simulink model "ModeloUnaOrugaFCVisibles"  (R2023b)
(part 3 of 16)

  Connection Label384/LConn1 -- Simscape Bus3/LConn5
  Connection Label309/LConn1 -- Simscape Bus2/LConn31
  Simscape Bus3/LConn16 -- Connection Label361/LConn1
  Connection Label364/LConn1 -- Simscape Bus3/LConn10
  Connection Label325/LConn1 -- Simscape Bus2/LConn17
  Connection Label342/LConn1 -- Simscape Bus3/LConn43
  Connection Label365/LConn1 -- Simscape Bus3/LConn28
  Connection Label345/LConn1 -- Simscape Bus3/LConn40
  Connection Label354/LConn1 -- Simscape Bus3/LConn31
  Connection Label315/LConn1 -- Simscape Bus2/LConn18
  Connection Label349/LConn1 -- Simscape Bus3/LConn36
  Connection Label338/LConn1 -- Simscape Bus2/LConn2
  Connection Label376/LConn1 -- Simscape Bus3/LConn25
  Simscape Bus3/LConn4 -- Connection Label381/LConn1
  Connection Label353/LConn1 -- Simscape Bus3/LConn32
  Simscape Bus2/LConn4 -- Connection Label337/LConn1
  Simscape Bus3/LConn24 -- Connection Label357/LConn1
  Connection Label323/LConn1 -- Simscape Bus2/LConn21
  Simscape Bus3/LConn8 -- Connection Label379/LConn1
  Connection Label331/LConn1 -- Simscape Bus2/LConn25
  Connection Label304/LConn1 -- Simscape Bus2/LConn36
  Simscape Bus2/LConn12 -- Connection Label318/LConn1
  Connection Label387/LConn1 -- Simscape Bus3/LConn47
  Connection Label308/LConn1 -- Simscape Bus2/LConn32
  Connection Label343/LConn1 -- Simscape Bus3/LConn42
  Simscape Bus3/LConn20 -- Connection Label359/LConn1
  Simscape Bus2/LConn8 -- Connection Label335/LConn1
  Connection Label341/LConn1 -- Simscape Bus2/LConn5
  Connection Label375/LConn1 -- Simscape Bus3/LConn27
  Connection Label317/LConn1 -- Simscape Bus2/LConn14
  Connection Label295/LConn1 -- Simscape Bus2/LConn45
  Simscape Bus3/LConn26 -- Connection Label366/LConn1
  Connection Label389/LConn1 -- Simscape Bus2/LConn49
  Simscape Bus2/LConn30 -- Connection Label310/LConn1
  Connection Label368/LConn1 -- Simscape Bus3/LConn21
  Connection Label356/LConn1 -- Simscape Bus3/LConn29
  Connection Label301/LConn1 -- Simscape Bus2/LConn39
  Connection Label367/LConn1 -- Simscape Bus3/LConn23
  Connection Label329/LConn1 -- Simscape Bus2/LConn9
  Connection Label298/LConn1 -- Simscape Bus2/LConn42
  Simscape Bus2/LConn22 -- Connection Label313/LConn1
  Connection Label322/LConn1 -- Simscape Bus2/LConn23
  Connection Label296/LConn1 -- Simscape Bus2/LConn44
  Connection Label374/LConn1 -- Simscape Bus3/LConn9
  Connection Label352/LConn1 -- Simscape Bus3/LConn33
  Connection Label378/LConn1 -- Simscape Bus3/LConn1
  Simscape Bus3/LConn22 -- Connection Label358/LConn1
  Simscape Bus3/RConn1 -- AAP/RConn1
  Connection Label385/LConn1 -- Simscape Bus3/LConn49
  Simscape Bus2/RConn1 -- AA/RConn1
  Revolute Joint34/LConn1 -- Pieza_Correa_61_RIGID/RConn1
  Revolute Joint43/LConn1 -- Pieza_Correa_52_RIGID/RConn1
  Revolute Joint47/LConn1 -- Pieza_Correa_74_RIGID/LConn1
  Revolute Joint13/LConn1 -- Pieza_Correa_88_RIGID/RConn1
  Revolute Joint31/LConn1 -- Pieza_Correa_64_RIGID/RConn1
  Revolute Joint10/LConn1 -- Pieza_Correa_85_RIGID/RConn1
  Revolute Joint40/RConn1 -- Pieza_Correa_56_RIGID/LConn1
  Revolute Joint6/RConn1 -- Pieza_Correa_82_RIGID/LConn1
  Revolute Joint7/LConn1 -- Pieza_Correa_82_RIGID/RConn1
  Revolute Joint3/LConn1 -- Pieza_Correa_78_RIGID1/RConn1
  Revolute Joint46/RConn1 -- Pieza_Correa_50_RIGID/LConn1
  Revolute Joint37/LConn1 -- Pieza_Correa_58_RIGID/RConn1
  Revolute Joint16/RConn1 -- Pieza_Correa_92_RIGID/LConn1
  Revolute Joint3/RConn1 -- Pieza_Correa_79_RIGID/LConn1
  Revolute Joint25/RConn1 -- Pieza_Correa_71_RIGID/LConn1
  Revolute Joint21/LConn1 -- Pieza_Correa_96_RIGID/RConn1
  Revolute Joint48/RConn1 -- Pieza_Correa_90_RIGID/LConn1
  Revolute Joint14/LConn1 -- Pieza_Correa_97_RIGID/RConn1
  Revolute Joint24/LConn1 -- Pieza_Correa_71_RIGID/RConn1
  Revolute Joint43/RConn1 -- Pieza_Correa_53_RIGID/LConn1
  Revolute Joint28/RConn1 -- Pieza_Correa_68_RIGID/LConn1
  Revolute Joint/LConn1 -- Pieza_Correa_1_RIGID/LConn2
  Revolute Joint23/LConn1 -- Pieza_Correa_72_RIGID/RConn1
  Revolute Joint12/RConn1 -- Pieza_Correa_88_RIGID/LConn1
  Revolute Joint15/LConn1 -- Pieza_Correa_90_RIGID/RConn1
  Revolute Joint21/RConn1 -- Pieza_Correa_97_RIGID/LConn1
  Revolute Joint22/LConn1 -- Pieza_Correa_75_RIGID/LConn1
  Revolute Joint5/RConn1 -- Pieza_Correa_81_RIGID/LConn1
  Revolute Joint46/LConn1 -- Pieza_Correa_1_RIGID/RConn3
  Revolute Joint2/RConn1 -- Pieza_Correa_78_RIGID1/LConn1
  Revolute Joint16/LConn1 -- Pieza_Correa_91_RIGID/RConn1
  Revolute Joint11/LConn1 -- Pieza_Correa_86_RIGID/RConn1
  Revolute Joint48/LConn1 -- Pieza_Correa_89_RIGID/RConn1
  Revolute Joint23/RConn1 -- Pieza_Correa_73_RIGID/LConn1
  Revolute Joint11/RConn1 -- Pieza_Correa_87_RIGID/LConn1
  Revolute Joint39/LConn1 -- Pieza_Correa_56_RIGID/RConn1
  Revolute Joint18/RConn1 -- Pieza_Correa_94_RIGID/LConn1
  Revolute Joint4/RConn1 -- Pieza_Correa_80_RIGID/LConn1
  Revolute Joint12/LConn1 -- Pieza_Correa_87_RIGID/RConn1
  Revolute Joint26/RConn1 -- Pieza_Correa_70_RIGID/LConn1
  Revolute Joint5/LConn1 -- Pieza_Correa_80_RIGID/RConn1
  Revolute Joint34/RConn1 -- Pieza_Correa_62_RIGID/LConn1
  Revolute Joint30/RConn1 -- Pieza_Correa_66_RIGID/LConn1
  Revolute Joint33/LConn1 -- Pieza_Correa_62_RIGID/RConn1
  Revolute Joint20/RConn1 -- Pieza_Correa_96_RIGID/LConn1
  Revolute Joint27/RConn1 -- Pieza_Correa_69_RIGID/LConn1
  Revolute Joint37/RConn1 -- Pieza_Correa_59_RIGID/LConn1
  Revolute Joint15/RConn1 -- Pieza_Correa_91_RIGID/LConn1
  Revolute Joint19/LConn1 -- Pieza_Correa_94_RIGID/RConn1
  Revolute Joint1/RConn1 -- Pieza_Correa_77_RIGID/LConn1
  Revolute Joint8/LConn1 -- Pieza_Correa_83_RIGID/RConn1
  Revolute Joint20/LConn1 -- Pieza_Correa_95_RIGID/RConn1
  Revolute Joint24/RConn1 -- Pieza_Correa_72_RIGID/LConn1
  Revolute Joint7/RConn1 -- Pieza_Correa_83_RIGID/LConn1
  Revolute Joint41/LConn1 -- Pieza_Correa_54_RIGID/RConn1
  Revolute Joint29/RConn1 -- Pieza_Correa_67_RIGID/LConn1
  Revolute Joint17/LConn1 -- Pieza_Correa_92_RIGID/RConn1
  Pieza_Correa_73_RIGID/RConn1 -- Revolute Joint47/RConn1
  Revolute Joint36/RConn1 -- Pieza_Correa_60_RIGID/LConn1
  Revolute Joint13/RConn1 -- Pieza_Correa_89_RIGID/LConn1
  Revolute Joint8/RConn1 -- Pieza_Correa_84_RIGID/LConn1
  Revolute Joint22/RConn1 -- Pieza_Correa_74_RIGID/RConn1
  Revolute Joint26/LConn1 -- Pieza_Correa_69_RIGID/RConn1
  Revolute Joint10/RConn1 -- Pieza_Correa_86_RIGID/LConn1
  Revolute Joint40/LConn1 -- Pieza_Correa_55_RIGID/RConn1
  Revolute Joint36/LConn1 -- Pieza_Correa_59_RIGID/RConn1
  Revolute Joint39/RConn1 -- Pieza_Correa_57_RIGID/LConn1
  Revolute Joint14/RConn1 -- Pieza_Correa_75_RIGID/RConn1
  Revolute Joint35/LConn1 -- Pieza_Correa_60_RIGID/RConn1
  Revolute Joint33/RConn1 -- Pieza_Correa_63_RIGID/LConn1
  Revolute Joint38/LConn1 -- Pieza_Correa_57_RIGID/RConn1
  Revolute Joint31/RConn1 -- Pieza_Correa_65_RIGID/LConn1
  Revolute Joint38/RConn1 -- Pieza_Correa_58_RIGID/LConn1
  Revolute Joint42/RConn1 -- Pieza_Correa_54_RIGID/LConn1
  Revolute Joint35/RConn1 -- Pieza_Correa_61_RIGID/LConn1
  Revolute Joint32/RConn1 -- Pieza_Correa_64_RIGID/LConn1
  Revolute Joint45/LConn1 -- Pieza_Correa_50_RIGID/RConn1
  Revolute Joint44/RConn1 -- Pieza_Correa_52_RIGID/LConn1
  Revolute Joint17/RConn1 -- Pieza_Correa_93_RIGID/LConn1
  Revolute Joint2/LConn1 -- Pieza_Correa_77_RIGID/RConn1
  Revolute Joint6/LConn1 -- Pieza_Correa_81_RIGID/RConn1
  Revolute Joint29/LConn1 -- Pieza_Correa_66_RIGID/RConn1
  Revolute Joint28/LConn1 -- Pieza_Correa_67_RIGID/RConn1
  Revolute Joint4/LConn1 -- Pieza_Correa_79_RIGID/RConn1
  Revolute Joint/RConn1 -- Pieza_Correa_76_RIGID/LConn1
  Revolute Joint9/RConn1 -- Pieza_Correa_85_RIGID/LConn1
  Revolute Joint19/RConn1 -- Pieza_Correa_95_RIGID/LConn1
  Revolute Joint27/LConn1 -- Pieza_Correa_68_RIGID/RConn1
  Revolute Joint1/LConn1 -- Pieza_Correa_76_RIGID/RConn1
  Revolute Joint25/LConn1 -- Pieza_Correa_70_RIGID/RConn1
  Revolute Joint30/LConn1 -- Pieza_Correa_65_RIGID/RConn1
  Revolute Joint42/LConn1 -- Pieza_Correa_53_RIGID/RConn1
  Revolute Joint18/LConn1 -- Pieza_Correa_93_RIGID/RConn1
  Revolute Joint9/LConn1 -- Pieza_Correa_84_RIGID/RConn1
  Revolute Joint45/RConn1 -- Pieza_Correa_51_RIGID/LConn1
  Revolute Joint32/LConn1 -- Pieza_Correa_63_RIGID/RConn1
  Revolute Joint44/LConn1 -- Pieza_Correa_51_RIGID/RConn1
  Pieza_Correa_1_RIGID/RConn1 -- Connection Label8/LConn1
  Pieza_Correa_1_RIGID/RConn2 -- Connection Label12/LConn1
  Connection Label79/LConn1 -- Pieza_Correa_92_RIGID/LConn2
  Connection Label76/LConn1 -- Pieza_Correa_92_RIGID/LConn3
  Pieza_Correa_93_RIGID/LConn2 -- Connection Label83/LConn1
  Connection Label80/LConn1 -- Pieza_Correa_93_RIGID/LConn3
  Pieza_Correa_94_RIGID/LConn3 -- Connection Label84/LConn1
  Pieza_Correa_94_RIGID/LConn2 -- Connection Label87/LConn1
  Pieza_Correa_95_RIGID/LConn3 -- Connection Label88/LConn1
  Pieza_Correa_95_RIGID/LConn2 -- Connection Label91/LConn1
  Pieza_Correa_96_RIGID/LConn3 -- Connection Label92/LConn1
  Pieza_Correa_96_RIGID/LConn2 -- Connection Label95/LConn1
  Pieza_Correa_75_RIGID/LConn2 -- Connection Label100/LConn1
  Pieza_Correa_75_RIGID/LConn3 -- Connection Label103/LConn1
  Pieza_Correa_74_RIGID/LConn2 -- Connection Label104/LConn1
  Pieza_Correa_74_RIGID/LConn3 -- Connection Label107/LConn1
  Pieza_Correa_73_RIGID/LConn3 -- Connection Label108/LConn1
  Pieza_Correa_73_RIGID/LConn2 -- Connection Label111/LConn1
  Pieza_Correa_72_RIGID/LConn3 -- Connection Label112/LConn1
  Pieza_Correa_72_RIGID/LConn2 -- Connection Label115/LConn1
  Pieza_Correa_71_RIGID/LConn3 -- Connection Label116/LConn1
  Pieza_Correa_71_RIGID/LConn2 -- Connection Label119/LConn1
  Pieza_Correa_70_RIGID/LConn3 -- Connection Label120/LConn1
  Pieza_Correa_70_RIGID/LConn2 -- Connection Label123/LConn1
  Pieza_Correa_69_RIGID/LConn3 -- Connection Label124/LConn1
  Pieza_Correa_69_RIGID/LConn2 -- Connection Label127/LConn1
  Pieza_Correa_68_RIGID/LConn3 -- Connection Label128/LConn1
  Pieza_Correa_68_RIGID/LConn2 -- Connection Label131/LConn1
  Pieza_Correa_67_RIGID/LConn3 -- Connection Label132/LConn1
  Pieza_Correa_67_RIGID/LConn2 -- Connection Label135/LConn1
  Pieza_Correa_66_RIGID/LConn3 -- Connection Label136/LConn1
  Pieza_Correa_66_RIGID/LConn2 -- Connection Label139/LConn1
  Pieza_Correa_65_RIGID/LConn3 -- Connection Label140/LConn1
  Pieza_Correa_65_RIGID/LConn2 -- Connection Label143/LConn1
  Pieza_Correa_64_RIGID/LConn3 -- Connection Label144/LConn1
  Pieza_Correa_64_RIGID/LConn2 -- Connection Label147/LConn1
  Pieza_Correa_63_RIGID/LConn3 -- Connection Label148/LConn1
  Pieza_Correa_63_RIGID/LConn2 -- Connection Label151/LConn1
  Pieza_Correa_62_RIGID/LConn3 -- Connection Label152/LConn1
  Pieza_Correa_62_RIGID/LConn2 -- Connection Label155/LConn1
  Pieza_Correa_61_RIGID/LConn3 -- Connection Label156/LConn1
  Pieza_Correa_61_RIGID/LConn2 -- Connection Label159/LConn1
  Pieza_Correa_60_RIGID/LConn3 -- Connection Label160/LConn1
  Pieza_Correa_60_RIGID/LConn2 -- Connection Label163/LConn1
  Pieza_Correa_59_RIGID/LConn3 -- Connection Label164/LConn1
  Pieza_Correa_59_RIGID/LConn2 -- Connection Label167/LConn1
  Pieza_Correa_58_RIGID/LConn3 -- Connection Label168/LConn1
  Pieza_Correa_58_RIGID/LConn2 -- Connection Label171/LConn1
  Pieza_Correa_57_RIGID/LConn3 -- Connection Label172/LConn1
  Pieza_Correa_57_RIGID/LConn2 -- Connection Label175/LConn1
  Pieza_Correa_56_RIGID/LConn3 -- Connection Label176/LConn1
  Pieza_Correa_56_RIGID/LConn2 -- Connection Label179/LConn1
  Pieza_Correa_55_RIGID/LConn3 -- Connection Label180/LConn1
  Pieza_Correa_55_RIGID/LConn2 -- Connection Label183/LConn1
  Pieza_Correa_54_RIGID/LConn3 -- Connection Label184/LConn1
  Pieza_Correa_54_RIGID/LConn2 -- Connection Label187/LConn1
  Pieza_Correa_53_RIGID/LConn3 -- Connection Label188/LConn1
  Pieza_Correa_53_RIGID/LConn2 -- Connection Label191/LConn1
  Pieza_Correa_52_RIGID/LConn3 -- Connection Label192/LConn1
  Pieza_Correa_52_RIGID/LConn2 -- Connection Label195/LConn1
  Pieza_Correa_51_RIGID/LConn3 -- Connection Label196/LConn1
  Pieza_Correa_51_RIGID/LConn2 -- Connection Label199/LConn1
  Pieza_Correa_50_RIGID/LConn3 -- Connection Label200/LConn1
  Pieza_Correa_50_RIGID/LConn2 -- Connection Label203/LConn1
  Revolute Joint41/RConn1 -- Pieza_Correa_55_RIGID/LConn1
